simulink model "GasTurbine_Dyn_Template_GPT_RLS_Blocks"  (Simulink 9.2)
settings: Solver=ode4  StartTime=0.0  StopTime=MWS.in.SimTime  FixedStep=MWS.Solve.T  RelTol=1e-3  EnableMultiTasking=on
PreLoadFcn:
  | tmats_rls_setup;
values from neighbouring files (symbols this model uses):
  MWS = tmats_gpt_setup()    [run_tmats_gpt.m]
undefined symbols (not defined in the file or in its folder): RLS, stripchar_TMATS
libraries: simulink x7, Lib_Solve_ModelSource_TMATS x2, Lib_Cntrl_FirstOrderSensor_TMATS x1, Lib_Turbo_Ambient_TMATS x1, Lib_Turbo_Burner_TMATS x1, Lib_Turbo_Compressor_TMATS x1, Lib_Turbo_Duct_TMATS x1, Lib_Turbo_Inlet_TMATS x1, Lib_Turbo_Nozzle_TMATS x1, Lib_Turbo_Shaft_TMATS x1, Lib_Turbo_Turbine_TMATS x1, Lib_Solve_IterNRSolverJC_TMATS x1
Description:
  | Basic-block RLS ARX(5,5,1) fuel-to-acceleration observer. No estimator S-function or MATLAB Function.
settings Model: Creator=jwchapm2  LastModifiedBy=volka
settings DataIOCC: SignalLoggingSaveFormat=Dataset  SignalLoggingName=SimulationOutput
settings OptimizationCC: BlockReduction=off  DefaultParameterBehavior=Inlined  BufferReuse=off  ExpressionDepthLimit=2147483647
settings DebuggingCC: SolverPrmCheckMsg=warning  FcnCallInpInsideContextMsg=error
settings GRTTargetCC: CombineOutputUpdateFcns=on  GRTInterface=off

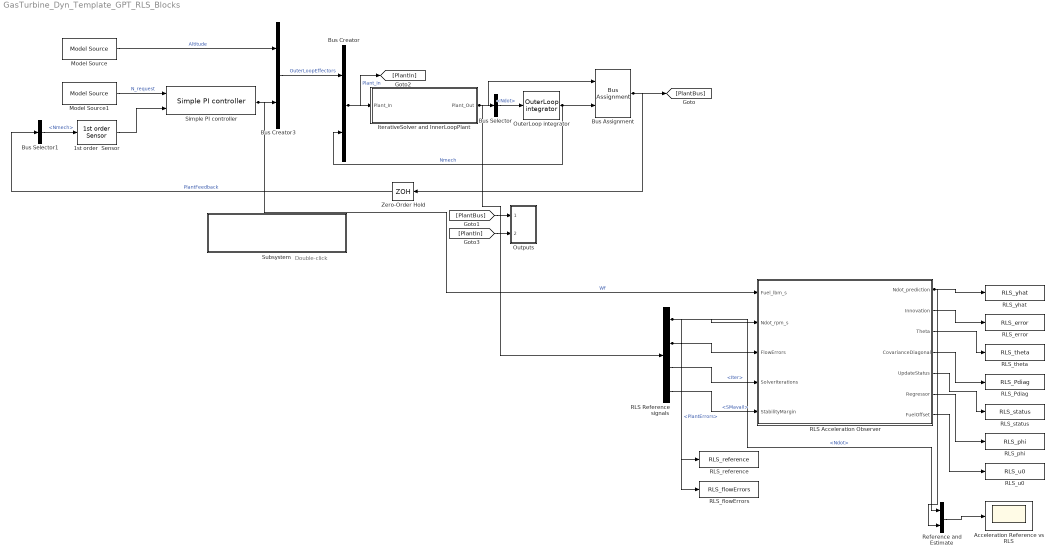
== system GasTurbine_Dyn_Template_GPT_RLS_Blocks ==
  note: Double-click
  1st order  Sensor : Lib_Cntrl_FirstOrderSensor_TMATS/1st order  Sensor  IC_M=MWS.Solve.N_IC  Sen_Max_M=20000  Sen_Min_M=0  Gain_M=1  Tau_M=0.05  GN_EN_M=off  GN_NST_M=MWS.Solve.T  GN_C_M=1  GN_MinNoise_M=0.3  F_Gain_M=1  F_Drift_M=0
  Acceleration Reference vs RLS : Scope
  Bus Assignment : BusAssignment  AssignedSignals=PlantBus.Nmech
  Bus Creator : BusCreator  Inputs=2
  Bus Creator3 : BusCreator  Inputs=2
  Bus Selector : BusSelector  OutputSignals=PlantBus.Ndot
  Bus Selector1 : BusSelector  OutputSignals=PlantBus.Nmech
  IterativeSolver and InnerLoopPlant : Subsystem
  Model Source : Lib_Solve_ModelSource_TMATS/Model Source  T_vec_M=MWS.in.t_vec  input_array_M=MWS.in.Alt
  Model Source1 : Lib_Solve_ModelSource_TMATS/Model Source  T_vec_M=MWS.in.t_vec  input_array_M=MWS.in.Ndmd
  OuterLoop integrator : Lib_Solve_OuterLoopIntegrator_TMATS/OuterLoop integrator  OL_IC_M=MWS.Solve.N_IC
  Outputs : Subsystem
  RLS Acceleration Observer : Subsystem
  RLS Reference signals : BusSelector  OutputSignals=PlantBus.Ndot,PlantErrors,PlantBus.Iter,PlantBus.C_Data.SMavail
  RLS_Pdiag : ToWorkspace  VariableName=RLS_Pdiag  SaveFormat=Timeseries  SampleTime=-1
  RLS_error : ToWorkspace  VariableName=RLS_error  SaveFormat=Timeseries  SampleTime=-1
  RLS_flowErrors : ToWorkspace  VariableName=RLS_flowErrors  SaveFormat=Timeseries  SampleTime=-1
  RLS_phi : ToWorkspace  VariableName=RLS_phi  SaveFormat=Timeseries  SampleTime=-1
  RLS_reference : ToWorkspace  VariableName=RLS_reference  SaveFormat=Timeseries  SampleTime=-1
  RLS_status : ToWorkspace  VariableName=RLS_status  SaveFormat=Timeseries  SampleTime=-1
  RLS_theta : ToWorkspace  VariableName=RLS_theta  SaveFormat=Timeseries  SampleTime=-1
  RLS_u0 : ToWorkspace  VariableName=RLS_u0  SaveFormat=Timeseries  SampleTime=-1
  RLS_yhat : ToWorkspace  VariableName=RLS_yhat  SaveFormat=Timeseries  SampleTime=-1
  Reference and Estimate : Mux  Inputs=2
  Simple PI controller : Lib_Cntrl_SimplePIcontroller_TMATS/Simple PI controller  Kp_M=0.05/2  Ki_M=0.1/2  PI_IC_M=3
  Subsystem : Subsystem
      settings: OpenFcn=run('PlotDynData.m')
      mask Display: fprintf('Plot Outputs')
  Zero-Order Hold : ZeroOrderHold  SampleTime=MWS.Solve.T
  wires:
  Bus Selector1/1 -> 1st order  Sensor/1  "<Nmech>"
  Reference and Estimate/1 -> Acceleration Reference vs RLS/1
  IterativeSolver and InnerLoopPlant/1(Plant_Out) -> Bus Assignment/1, Bus Selector/1, RLS Reference signals/1
  OuterLoop integrator/1 -> Bus Assignment/2, Bus Creator/2  "Nmech"
  Bus Creator3/1 -> Bus Creator/1  "OuterLoopEffectors"
  Model Source/1 -> Bus Creator3/1  "Altitude"
  Simple PI controller/1 -> Bus Creator3/2, RLS Acceleration Observer/1(Fuel_lbm_s)  "Wf"
  Zero-Order Hold/1 -> Bus Selector1/1  "PlantFeedback"
  Bus Assignment/1 -> [PlantBus], Zero-Order Hold/1
  Bus Creator/1 -> [PlantIn], IterativeSolver and InnerLoopPlant/1(Plant_In)  "Plant_In"
  Bus Selector/1 -> OuterLoop integrator/1  "<Ndot>"
  [PlantBus] -> Outputs/1(PlantOut)
  [PlantIn] -> Outputs/2(PlantIn)
  RLS Reference signals/1 -> RLS Acceleration Observer/2(Ndot_rpm_s), RLS_reference/1, Reference and Estimate/1  "<Ndot>"
  RLS Reference signals/2 -> RLS Acceleration Observer/3(FlowErrors), RLS_flowErrors/1  "<PlantErrors>"
  RLS Reference signals/3 -> RLS Acceleration Observer/4(SolverIterations)  "<Iter>"
  RLS Reference signals/4 -> RLS Acceleration Observer/5(StabilityMargin)  "<SMavail>"
  RLS Acceleration Observer/4(CovarianceDiagonal) -> RLS_Pdiag/1
  RLS Acceleration Observer/2(Innovation) -> RLS_error/1
  RLS Acceleration Observer/6(Regressor) -> RLS_phi/1
  RLS Acceleration Observer/5(UpdateStatus) -> RLS_status/1
  RLS Acceleration Observer/3(Theta) -> RLS_theta/1
  RLS Acceleration Observer/7(FuelOffset) -> RLS_u0/1
  RLS Acceleration Observer/1(Ndot_prediction) -> RLS_yhat/1, Reference and Estimate/2
  Model Source1/1 -> Simple PI controller/1  "N_request"
  1st order  Sensor/1 -> Simple PI controller/2

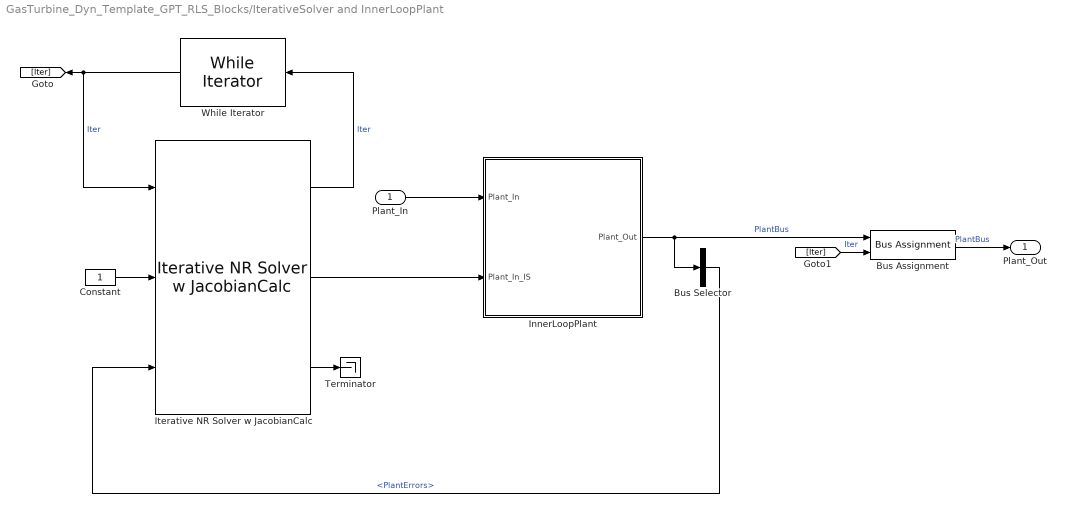
== system GasTurbine_Dyn_Template_GPT_RLS_Blocks/IterativeSolver and InnerLoopPlant ==
  Plant_In : Inport
  Bus Assignment : BusAssignment  AssignedSignals=PlantBus.Iter
  Bus Selector : BusSelector  OutputSignals=PlantErrors
  Constant : Constant
  InnerLoopPlant : Subsystem
  Iterative NR Solver w JacobianCalc : Lib_Solve_IterNRSolverJC_TMATS/Iterative NR Solver w JacobianCalc  SJac_Per_M=MWS.Solve.J_Calc_Per  SNR_IC_M=MWS.Solve.NR_IC  SNR_DX_M=MWS.Solve.NR_dx  SNR_Mx_M=100000  SNR_Mn_M=0.0001  SJacobianAttempts_M=MWS.Solve.NR_Jac_Re  Cond_Limits_M=MWS.Solve.C_Lim
  Terminator : Terminator
  While Iterator : WhileIterator  MaxIters=MWS.Solve.Max_Iter  WhileBlockType=do-while  ShowIterationPort=on
  Plant_Out : Outport
  wires:
  Plant_In/1 -> InnerLoopPlant/1(Plant_In)
  Bus Selector/1 -> Iterative NR Solver w JacobianCalc/3  "<PlantErrors>"
  While Iterator/1 -> [Iter], Iterative NR Solver w JacobianCalc/1  "Iter"
  InnerLoopPlant/1(Plant_Out) -> Bus Assignment/1, Bus Selector/1  "PlantBus"
  Iterative NR Solver w JacobianCalc/2 -> InnerLoopPlant/2(Plant_In_IS)
  Iterative NR Solver w JacobianCalc/1 -> While Iterator/1  "Iter"
  Iterative NR Solver w JacobianCalc/3 -> Terminator/1
  Constant/1 -> Iterative NR Solver w JacobianCalc/2
  [Iter] -> Bus Assignment/2  "Iter"
  Bus Assignment/1 -> Plant_Out/1  "PlantBus"

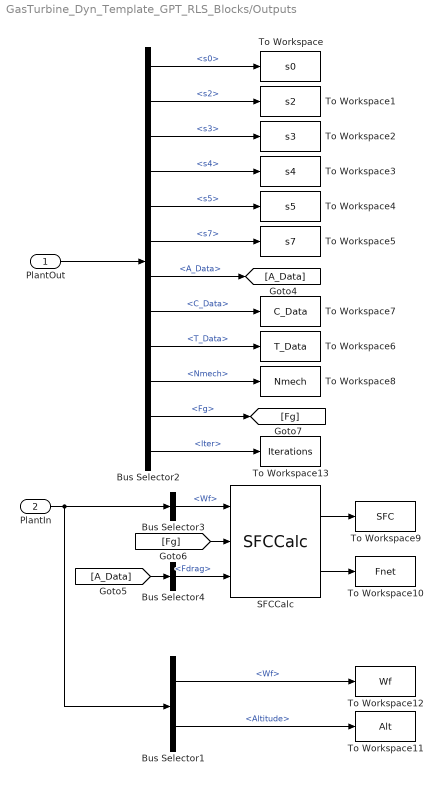
== system GasTurbine_Dyn_Template_GPT_RLS_Blocks/Outputs ==
  PlantOut : Inport
  PlantIn : Inport  Port=2
  Bus Selector1 : BusSelector  OutputSignals=OuterLoopEffectors.Wf,OuterLoopEffectors.Altitude
  Bus Selector2 : BusSelector  OutputSignals=PlantBus.s0,PlantBus.s2,PlantBus.s3,PlantBus.s4,PlantBus.s5,PlantBus.s7,PlantBus.A_Data,PlantBus.C_Data,PlantBus.T_Data,PlantBus.Nmech,PlantBus.Fg,PlantBus.Iter
  Bus Selector3 : BusSelector  OutputSignals=OuterLoopEffectors.Wf
  Bus Selector4 : BusSelector  OutputSignals=Fdrag
  SFCCalc : Lib_Turbo_SFCCalc_TMATS/SFCCalc
  To Workspace : ToWorkspace  VariableName=s0  SaveFormat=Timeseries  SampleTime=-1
  To Workspace1 : ToWorkspace  VariableName=s2  SaveFormat=Timeseries  SampleTime=-1
  To Workspace10 : ToWorkspace  VariableName=Fnet  SaveFormat=Timeseries  SampleTime=-1
  To Workspace11 : ToWorkspace  VariableName=Alt  SaveFormat=Timeseries  SampleTime=-1
  To Workspace12 : ToWorkspace  VariableName=Wf  SaveFormat=Timeseries  SampleTime=-1
  To Workspace13 : ToWorkspace  VariableName=Iterations  SaveFormat=Timeseries  SampleTime=-1
  To Workspace2 : ToWorkspace  VariableName=s3  SaveFormat=Timeseries  SampleTime=-1
  To Workspace3 : ToWorkspace  VariableName=s4  SaveFormat=Timeseries  SampleTime=-1
  To Workspace4 : ToWorkspace  VariableName=s5  SaveFormat=Timeseries  SampleTime=-1
  To Workspace5 : ToWorkspace  VariableName=s7  SaveFormat=Timeseries  SampleTime=-1
  To Workspace6 : ToWorkspace  VariableName=T_Data  SaveFormat=Timeseries  SampleTime=-1
  To Workspace7 : ToWorkspace  VariableName=C_Data  SaveFormat=Timeseries  SampleTime=-1
  To Workspace8 : ToWorkspace  VariableName=Nmech  SaveFormat=Timeseries  SampleTime=-1
  To Workspace9 : ToWorkspace  VariableName=SFC  SaveFormat=Timeseries  SampleTime=-1
  wires:
  SFCCalc/2 -> To Workspace10/1
  Bus Selector2/5 -> To Workspace4/1  "<s5>"
  SFCCalc/1 -> To Workspace9/1
  Bus Selector3/1 -> SFCCalc/1  "<Wf>"
  Bus Selector2/6 -> To Workspace5/1  "<s7>"
  Bus Selector2/11 -> [Fg]  "<Fg>"
  Bus Selector4/1 -> SFCCalc/3  "<Fdrag>"
  Bus Selector2/10 -> To Workspace8/1  "<Nmech>"
  Bus Selector2/1 -> To Workspace/1  "<s0>"
  Bus Selector2/3 -> To Workspace2/1  "<s3>"
  Bus Selector2/8 -> To Workspace7/1  "<C_Data>"
  Bus Selector2/9 -> To Workspace6/1  "<T_Data>"
  Bus Selector2/7 -> [A_Data]  "<A_Data>"
  PlantOut/1 -> Bus Selector2/1
  [Fg] -> SFCCalc/2
  Bus Selector2/2 -> To Workspace1/1  "<s2>"
  Bus Selector2/4 -> To Workspace3/1  "<s4>"
  PlantIn/1 -> Bus Selector1/1, Bus Selector3/1
  [A_Data] -> Bus Selector4/1
  Bus Selector1/1 -> To Workspace12/1  "<Wf>"
  Bus Selector1/2 -> To Workspace11/1  "<Altitude>"
  Bus Selector2/12 -> To Workspace13/1  "<Iter>"

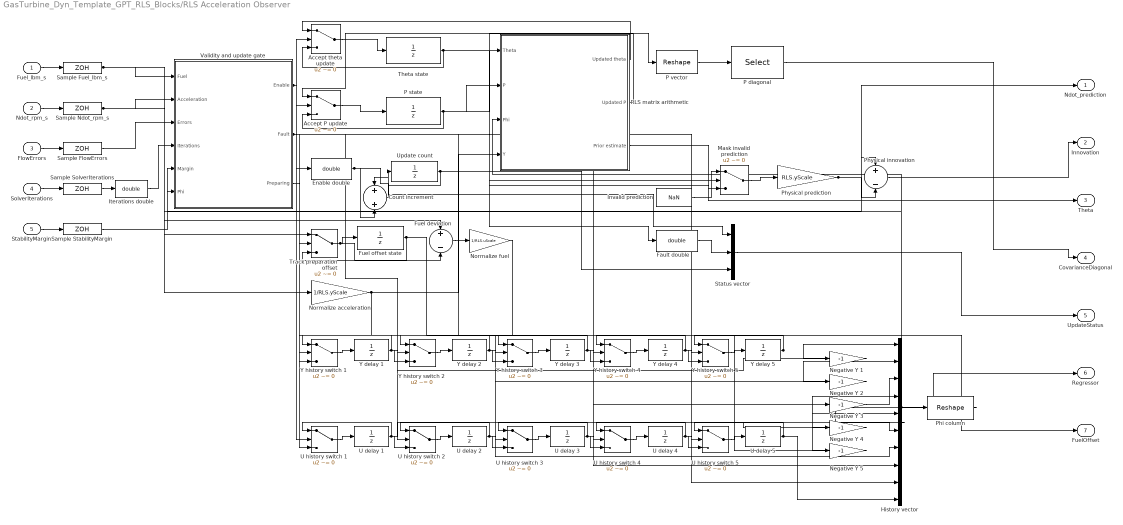
== system GasTurbine_Dyn_Template_GPT_RLS_Blocks/RLS Acceleration Observer ==
  Fuel_lbm_s : Inport
  Ndot_rpm_s : Inport  Port=2
  FlowErrors : Inport  Port=3
  SolverIterations : Inport  Port=4
  StabilityMargin : Inport  Port=5
  Accept P update : Switch  Criteria=u2 ~= 0
  Accept theta update : Switch  Criteria=u2 ~= 0
  Count increment : Sum
  Enable double : DataTypeConversion  OutDataTypeStr=double
  Fault double : DataTypeConversion  OutDataTypeStr=double
  Fuel deviation : Sum  Inputs=+-
  Fuel offset state : UnitDelay  InitialCondition=3  SampleTime=RLS.Ts
  History vector : Mux  Inputs=10
  Invalid prediction : Constant  Value=NaN
  Iterations double : DataTypeConversion  OutDataTypeStr=double
  Mask invalid prediction : Switch  Criteria=u2 ~= 0
  Negative Y {1..5} (5 alike) : Gain  Gain=-1
  Normalize acceleration : Gain  Gain=1/RLS.yScale
  Normalize fuel : Gain  Gain=1/RLS.uScale
  P diagonal : Selector  InputPortWidth=100  IndexOptions=Index vector (dialog)  Indices=1:11:100  OutputSizes=1
  P state : UnitDelay  InitialCondition=RLS.P0*eye(10)  SampleTime=RLS.Ts
  P vector : Reshape
  Phi column : Reshape  OutputDimensionality=Customize  OutputDimensions=[10 1]
  Physical innovation : Sum  Inputs=+-
  Physical prediction : Gain  Gain=RLS.yScale
  RLS matrix arithmetic : Subsystem
  Sample FlowErrors : ZeroOrderHold  SampleTime=RLS.Ts
  Sample Fuel_lbm_s : ZeroOrderHold  SampleTime=RLS.Ts
  Sample Ndot_rpm_s : ZeroOrderHold  SampleTime=RLS.Ts
  Sample SolverIterations : ZeroOrderHold  SampleTime=RLS.Ts
  Sample StabilityMargin : ZeroOrderHold  SampleTime=RLS.Ts
  Status vector : Mux  Inputs=3
  Theta state : UnitDelay  InitialCondition=zeros(10,1)  SampleTime=RLS.Ts
  Track preparation offset : Switch  Criteria=u2 ~= 0
  U delay {1..5} (5 alike) : UnitDelay  SampleTime=RLS.Ts
  U history switch {1..5} (5 alike) : Switch  Criteria=u2 ~= 0
  Update count : UnitDelay  SampleTime=RLS.Ts
  Validity and update gate : Subsystem
  Y delay {1..5} (5 alike) : UnitDelay  SampleTime=RLS.Ts
  Y history switch {1..5} (5 alike) : Switch  Criteria=u2 ~= 0
  Ndot_prediction : Outport
  Innovation : Outport  Port=2
  Theta : Outport  Port=3
  CovarianceDiagonal : Outport  Port=4
  UpdateStatus : Outport  Port=5
  Regressor : Outport  Port=6
  FuelOffset : Outport  Port=7
  wires:
  Fuel_lbm_s/1 -> Sample Fuel_lbm_s/1
  Ndot_rpm_s/1 -> Sample Ndot_rpm_s/1
  FlowErrors/1 -> Sample FlowErrors/1
  SolverIterations/1 -> Sample SolverIterations/1
  StabilityMargin/1 -> Sample StabilityMargin/1
  Sample SolverIterations/1 -> Iterations double/1
  Sample Fuel_lbm_s/1 -> Validity and update gate/1(Fuel), Track preparation offset/1, Fuel deviation/1
  Sample Ndot_rpm_s/1 -> Validity and update gate/2(Acceleration), Normalize acceleration/1, Physical innovation/1
  Sample FlowErrors/1 -> Validity and update gate/3(Errors)
  Iterations double/1 -> Validity and update gate/4(Iterations)
  Sample StabilityMargin/1 -> Validity and update gate/5(Margin)
  Validity and update gate/3(Preparing) -> Track preparation offset/2
  Fuel offset state/1 -> Track preparation offset/3, FuelOffset/1
  Track preparation offset/1 -> Fuel offset state/1, Fuel deviation/2
  Fuel deviation/1 -> Normalize fuel/1
  Y delay 1/1 -> Y history switch 1/1, Y history switch 2/3, Negative Y 1/1
  Validity and update gate/2(Fault) -> Y history switch 1/2, Y history switch 2/2, Y history switch 3/2, Y history switch 4/2, Y history switch 5/2, U history switch 1/2, U history switch 2/2, U history switch 3/2, U history switch 4/2, U history switch 5/2, Mask invalid prediction/2, Fault double/1
  Normalize acceleration/1 -> Y history switch 1/3, RLS matrix arithmetic/4(Y)
  Y history switch 1/1 -> Y delay 1/1
  Y delay 2/1 -> Y history switch 2/1, Y history switch 3/3, Negative Y 2/1
  Y history switch 2/1 -> Y delay 2/1
  Y delay 3/1 -> Y history switch 3/1, Y history switch 4/3, Negative Y 3/1
  Y history switch 3/1 -> Y delay 3/1
  Y delay 4/1 -> Y history switch 4/1, Y history switch 5/3, Negative Y 4/1
  Y history switch 4/1 -> Y delay 4/1
  Y delay 5/1 -> Y history switch 5/1, Negative Y 5/1
  Y history switch 5/1 -> Y delay 5/1
  U delay 1/1 -> U history switch 1/1, U history switch 2/3, History vector/6
  Normalize fuel/1 -> U history switch 1/3
  U history switch 1/1 -> U delay 1/1
  U delay 2/1 -> U history switch 2/1, U history switch 3/3, History vector/7
  U history switch 2/1 -> U delay 2/1
  U delay 3/1 -> U history switch 3/1, U history switch 4/3, History vector/8
  U history switch 3/1 -> U delay 3/1
  U delay 4/1 -> U history switch 4/1, U history switch 5/3, History vector/9
  U history switch 4/1 -> U delay 4/1
  U delay 5/1 -> U history switch 5/1, History vector/10
  U history switch 5/1 -> U delay 5/1
  Negative Y 1/1 -> History vector/1
  Negative Y 2/1 -> History vector/2
  Negative Y 3/1 -> History vector/3
  Negative Y 4/1 -> History vector/4
  Negative Y 5/1 -> History vector/5
  History vector/1 -> Phi column/1
  Phi column/1 -> Validity and update gate/6(Phi), RLS matrix arithmetic/3(Phi), Regressor/1
  Theta state/1 -> RLS matrix arithmetic/1(Theta), Accept theta update/3, Theta/1
  P state/1 -> RLS matrix arithmetic/2(P), Accept P update/3, P vector/1
  RLS matrix arithmetic/1(Updated theta) -> Accept theta update/1
  Validity and update gate/1(Enable) -> Accept theta update/2, Accept P update/2, Enable double/1
  RLS matrix arithmetic/2(Updated P) -> Accept P update/1
  Accept theta update/1 -> Theta state/1
  Accept P update/1 -> P state/1
  Invalid prediction/1 -> Mask invalid prediction/1
  RLS matrix arithmetic/3(Prior estimate) -> Mask invalid prediction/3
  Mask invalid prediction/1 -> Physical prediction/1
  Physical prediction/1 -> Physical innovation/2, Ndot_prediction/1
  P vector/1 -> P diagonal/1
  Update count/1 -> Count increment/1, Status vector/3
  Enable double/1 -> Count increment/2, Status vector/1
  Count increment/1 -> Update count/1
  Fault double/1 -> Status vector/2
  Physical innovation/1 -> Innovation/1
  P diagonal/1 -> CovarianceDiagonal/1
  Status vector/1 -> UpdateStatus/1

== system GasTurbine_Dyn_Template_GPT_RLS_Blocks/Subsystem ==

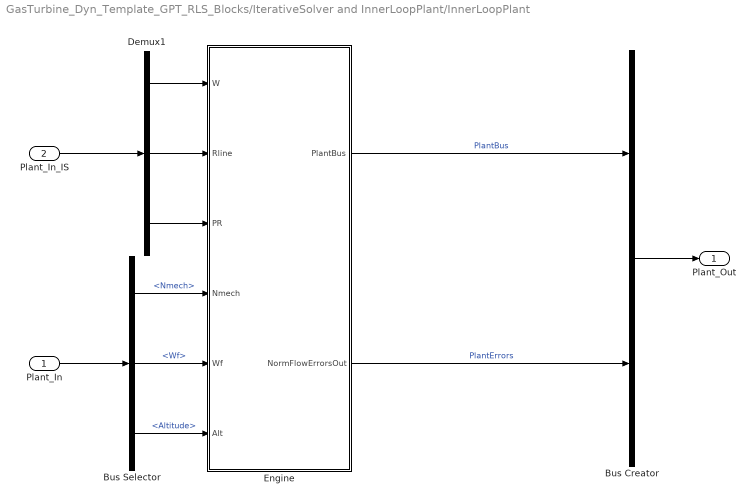
== system GasTurbine_Dyn_Template_GPT_RLS_Blocks/IterativeSolver and InnerLoopPlant/InnerLoopPlant ==
  Plant_In : Inport
  Plant_In_IS : Inport  Port=2
  Bus Selector : BusSelector  OutputSignals=Nmech,OuterLoopEffectors.Wf,OuterLoopEffectors.Altitude
  Bus Creator : BusCreator  Inputs=2
  Demux1 : Demux  Outputs=3
  Engine : Subsystem
  Plant_Out : Outport
  wires:
  Engine/1(PlantBus) -> Bus Creator/1  "PlantBus"
  Engine/2(NormFlowErrorsOut) -> Bus Creator/2  "PlantErrors"
  Bus Creator/1 -> Plant_Out/1
  Bus Selector/2 -> Engine/5(Wf)  "<Wf>"
  Bus Selector/1 -> Engine/4(Nmech)  "<Nmech>"
  Bus Selector/3 -> Engine/6(Alt)  "<Altitude>"
  Demux1/1 -> Engine/1(W)
  Demux1/2 -> Engine/2(Rline)
  Demux1/3 -> Engine/3(PR)
  Plant_In/1 -> Bus Selector/1
  Plant_In_IS/1 -> Demux1/1

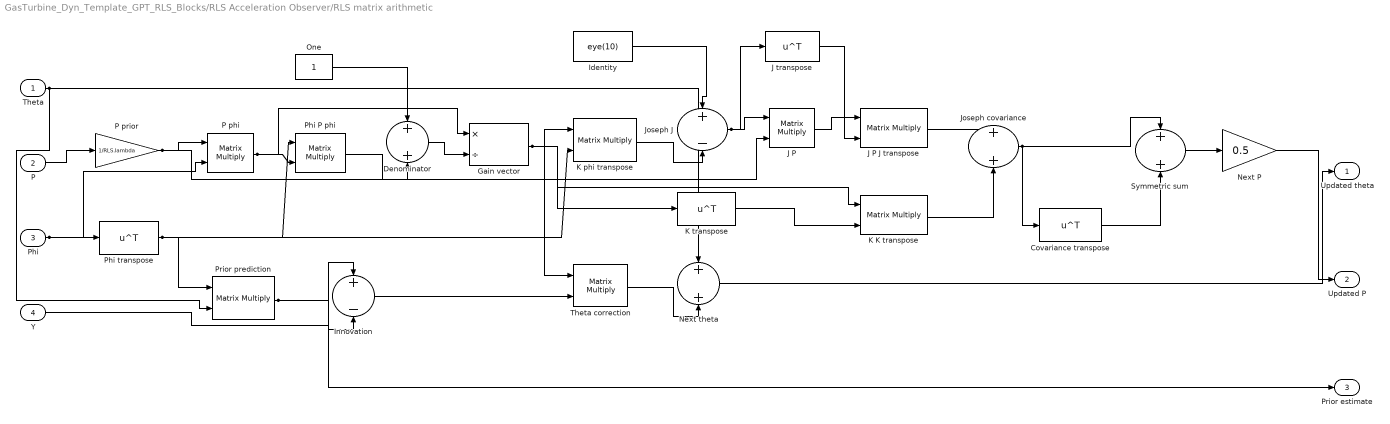
== system GasTurbine_Dyn_Template_GPT_RLS_Blocks/RLS Acceleration Observer/RLS matrix arithmetic ==
  Theta : Inport
  P : Inport  Port=2
  Phi : Inport  Port=3
  Y : Inport  Port=4
  Covariance transpose : Math  Operator=transpose  SaturateOnIntegerOverflow=on
  Denominator : Sum
  Gain vector : Product  Inputs=*/
  Identity : Constant  Value=eye(10)
  Innovation : Sum  Inputs=+-
  J P : Product  Inputs=**  Multiplication=Matrix(*)
  J P J transpose : Product  Inputs=**  Multiplication=Matrix(*)
  J transpose : Math  Operator=transpose  SaturateOnIntegerOverflow=on
  Joseph J : Sum  Inputs=+-
  Joseph covariance : Sum
  K K transpose : Product  Inputs=**  Multiplication=Matrix(*)
  K phi transpose : Product  Inputs=**  Multiplication=Matrix(*)
  K transpose : Math  Operator=transpose  SaturateOnIntegerOverflow=on
  Next P : Gain  Gain=0.5
  Next theta : Sum
  One : Constant
  P phi : Product  Inputs=**  Multiplication=Matrix(*)
  P prior : Gain  Gain=1/RLS.lambda
  Phi P phi : Product  Inputs=**  Multiplication=Matrix(*)
  Phi transpose : Math  Operator=transpose  SaturateOnIntegerOverflow=on
  Prior prediction : Product  Inputs=**  Multiplication=Matrix(*)
  Symmetric sum : Sum
  Theta correction : Product  Inputs=**  Multiplication=Matrix(*)
  Updated theta : Outport
  Updated P : Outport  Port=2
  Prior estimate : Outport  Port=3
  wires:
  P/1 -> P prior/1
  Phi/1 -> Phi transpose/1, P phi/2
  P prior/1 -> P phi/1, J P/2
  Phi transpose/1 -> Phi P phi/1, Prior prediction/1, K phi transpose/2
  P phi/1 -> Phi P phi/2, Gain vector/1
  One/1 -> Denominator/1
  Phi P phi/1 -> Denominator/2
  Denominator/1 -> Gain vector/2
  Theta/1 -> Prior prediction/2, Next theta/1
  Y/1 -> Innovation/1
  Prior prediction/1 -> Innovation/2, Prior estimate/1
  Gain vector/1 -> Theta correction/1, K phi transpose/1, K transpose/1, K K transpose/1
  Innovation/1 -> Theta correction/2
  Theta correction/1 -> Next theta/2
  Identity/1 -> Joseph J/1
  K phi transpose/1 -> Joseph J/2
  Joseph J/1 -> J P/1, J transpose/1
  J P/1 -> J P J transpose/1
  J transpose/1 -> J P J transpose/2
  K transpose/1 -> K K transpose/2
  J P J transpose/1 -> Joseph covariance/1
  K K transpose/1 -> Joseph covariance/2
  Joseph covariance/1 -> Covariance transpose/1, Symmetric sum/1
  Covariance transpose/1 -> Symmetric sum/2
  Symmetric sum/1 -> Next P/1
  Next theta/1 -> Updated theta/1
  Next P/1 -> Updated P/1

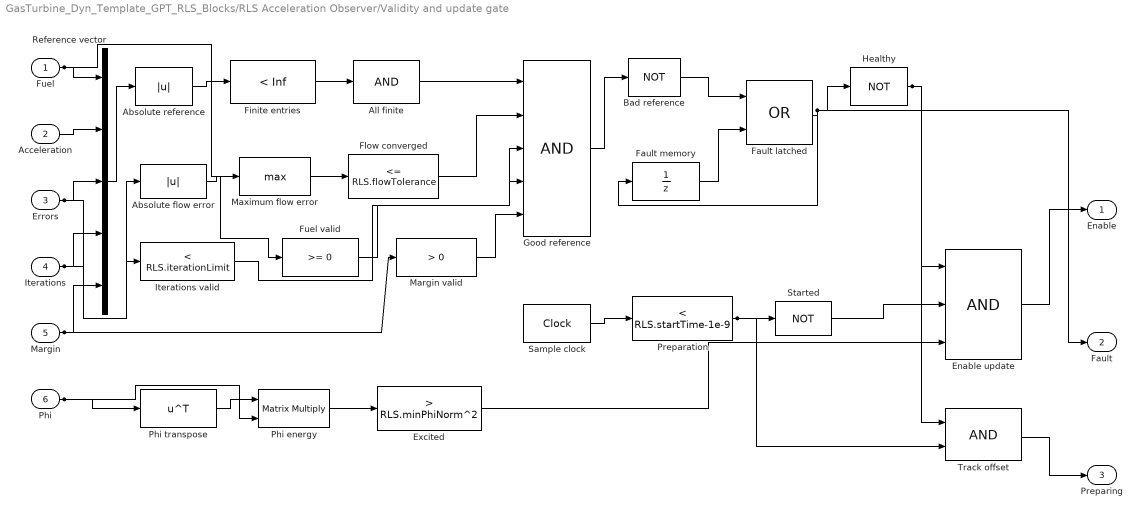
== system GasTurbine_Dyn_Template_GPT_RLS_Blocks/RLS Acceleration Observer/Validity and update gate ==
  Fuel : Inport
  Acceleration : Inport  Port=2
  Errors : Inport  Port=3
  Iterations : Inport  Port=4
  Margin : Inport  Port=5
  Phi : Inport  Port=6
  Absolute flow error : Abs
  Absolute reference : Abs
  All finite : Logic  Inputs=1  AllPortsSameDT=off  OutDataTypeStr=boolean
  Bad reference : Logic  Operator=NOT  AllPortsSameDT=off  OutDataTypeStr=boolean
  Enable update : Logic  Inputs=3  AllPortsSameDT=off  OutDataTypeStr=boolean
  Excited : simulink/Logic and Bit Operations/Compare To Constant  relop=>  const=RLS.minPhiNorm^2  OutDataTypeStr=boolean
  Fault latched : Logic  Operator=OR  AllPortsSameDT=off  OutDataTypeStr=boolean
  Fault memory : UnitDelay  InitialCondition=false  SampleTime=RLS.Ts
  Finite entries : simulink/Logic and Bit Operations/Compare To Constant  relop=<  const=Inf  OutDataTypeStr=boolean
  Flow converged : simulink/Logic and Bit Operations/Compare To Constant  relop=<=  const=RLS.flowTolerance  OutDataTypeStr=boolean
  Fuel valid : simulink/Logic and Bit Operations/Compare To Constant  relop=>=  const=0  OutDataTypeStr=boolean
  Good reference : Logic  Inputs=5  AllPortsSameDT=off  OutDataTypeStr=boolean
  Healthy : Logic  Operator=NOT  AllPortsSameDT=off  OutDataTypeStr=boolean
  Iterations valid : simulink/Logic and Bit Operations/Compare To Constant  relop=<  const=RLS.iterationLimit  OutDataTypeStr=boolean
  Margin valid : simulink/Logic and Bit Operations/Compare To Constant  relop=>  const=0  OutDataTypeStr=boolean
  Maximum flow error : MinMax  Function=max
  Phi energy : Product  Inputs=**  Multiplication=Matrix(*)
  Phi transpose : Math  Operator=transpose  SaturateOnIntegerOverflow=on
  Preparation : simulink/Logic and Bit Operations/Compare To Constant  relop=<  const=RLS.startTime-1e-9  OutDataTypeStr=boolean
  Reference vector : Mux  Inputs=5
  Sample clock : DigitalClock  SampleTime=RLS.Ts
  Started : Logic  Operator=NOT  AllPortsSameDT=off  OutDataTypeStr=boolean
  Track offset : Logic  AllPortsSameDT=off  OutDataTypeStr=boolean
  Enable : Outport
  Fault : Outport  Port=2
  Preparing : Outport  Port=3
  wires:
  Fuel/1 -> Reference vector/1, Fuel valid/1
  Acceleration/1 -> Reference vector/2
  Errors/1 -> Reference vector/3, Absolute flow error/1
  Iterations/1 -> Reference vector/4, Iterations valid/1
  Margin/1 -> Reference vector/5, Margin valid/1
  Reference vector/1 -> Absolute reference/1
  Absolute reference/1 -> Finite entries/1
  Finite entries/1 -> All finite/1
  Absolute flow error/1 -> Maximum flow error/1
  Maximum flow error/1 -> Flow converged/1
  All finite/1 -> Good reference/1
  Flow converged/1 -> Good reference/2
  Iterations valid/1 -> Good reference/3
  Fuel valid/1 -> Good reference/4
  Margin valid/1 -> Good reference/5
  Good reference/1 -> Bad reference/1
  Bad reference/1 -> Fault latched/1
  Fault memory/1 -> Fault latched/2
  Fault latched/1 -> Fault memory/1, Healthy/1, Fault/1
  Sample clock/1 -> Preparation/1
  Preparation/1 -> Started/1, Track offset/2
  Phi/1 -> Phi transpose/1, Phi energy/2
  Phi transpose/1 -> Phi energy/1
  Phi energy/1 -> Excited/1
  Healthy/1 -> Enable update/1, Track offset/1
  Started/1 -> Enable update/2
  Excited/1 -> Enable update/3
  Enable update/1 -> Enable/1
  Track offset/1 -> Preparing/1

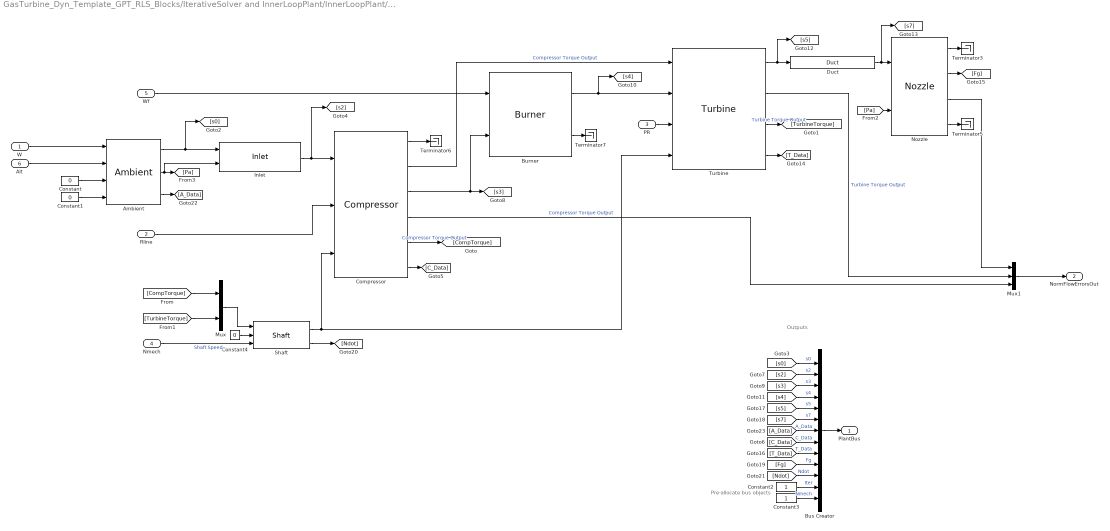
== system GasTurbine_Dyn_Template_GPT_RLS_Blocks/IterativeSolver and InnerLoopPlant/InnerLoopPlant/Engine ==
  note: Pre-allocate bus objects
  note: Outputs
  W : Inport
  Rline : Inport  Port=2
  PR : Inport  Port=3
  Nmech : Inport  Port=4
  Wf : Inport  Port=5
  Alt : Inport  Port=6
  Ambient : Lib_Turbo_Ambient_TMATS/Ambient  X_A_AltVec_M=5000*[-1 0 1 2 3 4 5 6 7 8 9 10 12 14 16]  T_A_TsVec_M=[536.51 518.67 500.84 483.03 465.22 447.41 429.62 411.84 394.06 389.97 389.97 389.97 389.97 392.25 397.69]  T_A_PsVec_M=[17.554 14.696 12.228 10.108 8.297 6.759 5.461 4.373 3.468 2.73 2.149 1.692 1.049 0.651 0.406]  AFARc_M=0  X_A_FARVec_M=[0; 0.0050; 0.0100; 0.0150; 0.0200; 0.0250; 0.0300]  T_A_RtArray_M="[0.0686;    0.0686;    0.0686;    0.0686;    0.0686;    0.0686;    0.0686]"  Y_A_TVec_M=[300 10000]  T_A_gammaArray_M=[ 1.4 1.4 1.4 1.4 1.4 1.4 1.4; 1.4 1.4 1.4 1.4 1.4 1.4 1.4]
  Burner : Lib_Turbo_Burner_TMATS/Burner  LHVEn_M=on  LHV_M=MWS.Burner.LHV  Eff_M=1  hFuel_M=-1200  dPnormBurner_M=MWS.Burner.dP
  Bus Creator : BusCreator  Inputs=13
  Compressor : Lib_Turbo_Compressor_TMATS/Compressor  X_C_RlineVec_M=MWS.HPC.RlineVec  Z_C_AlphaVec_M=1  Y_C_Map_NcVec_M=MWS.HPC.NcVec  T_C_Map_WcArray_M=MWS.HPC.WcArray  T_C_Map_PRArray_M=MWS.HPC.PRArray  T_C_Map_EffArray_M=MWS.HPC.EffArray  s_C_Nc_M=MWS.HPC.s_Nc  s_C_Wc_M=MWS.HPC.s_Wc  s_C_PR_M=MWS.HPC.s_PR  s_C_Eff_M=MWS.HPC.s_eff  SL_M=off  Scale_M=none  CBLDEN_M=off  C_CBD_M=0  C_CBFht_M=0.5  C_CBFPt_M=0.5  FBLDEN_M=off  C_FBD_M=0  C_BFht_M=0.5  C_BFPt_M=0.5  DefSMEn_M=off  SMNEn_M=off  SRline_M=1  X_C_Map_WcSurgeVec_M=MWS.HPC.WcMapSurge  T_C_Map_PRSurgeVec_M=MWS.HPC.PRMapSurge  iDesign_M=2  NcDes_M=10000  EffDes_M=0.85  PRDes_M=20  RlineDes_M=2  FVar_M=strcat('iDes_',stripchar_TMATS(gcb),'.bin')  BlkNm_M=double(gcb)  HP_M=off
  Constant : Constant  Value=0
  Constant1 : Constant  Value=0
  Constant2 : Constant  OutDataTypeStr=int32
  Constant3 : Constant
  Constant4 : Constant  Value=0
  Duct : Lib_Turbo_Duct_TMATS/Duct  dP_M=MWS.Duct.dP
  Inlet : Lib_Turbo_Inlet_TMATS/Inlet  eRambase_M=MWS.Inlet.eRambase  X_eRamVec_M=[0 3]  T_eRamtbl_M=[1 1]
  Mux : Mux  Inputs=2
  Mux1 : Mux  Inputs=3
  Nozzle : Lib_Turbo_Nozzle_TMATS/Nozzle  SWType_M=Convergent  N_TArea_M=MWS.Noz.ATh  N_EArea_M=110.7  N_FL_M=MWS.Noz.LossPerc  X_N_TtVec2_M=MWS.Noz.TtVec  T_N_TGArray_M=MWS.Noz.TGArray  X_N_PEQPaVec_M=MWS.Noz.PeQPaVec  T_N_CdThArray_M=MWS.Noz.CdThArray  T_N_CvArray_M=MWS.Noz.CvArray  CfgEn_M=off  T_N_CfgArray_M=[1 1]  X_N_FARVec_M=MWS.Noz.FARVec  T_N_RtArray_M=MWS.Noz.RArray  Y_N_TtVec_M=MWS.Noz.TtVec  T_N_MAP_gammaArray_M=MWS.Noz.GArray  iDesign_M=2  WDes_M=100  FVar_M=strcat('iDes_',stripchar_TMATS(gcb),'.bin')
  Shaft : Lib_Turbo_Shaft_TMATS/Shaft  Shaft_Inertia_M=MWS.Shaft.N_I
  Terminator{3,5..7} (4 alike) : Terminator
  Turbine : Lib_Turbo_Turbine_TMATS/Turbine  X_T_Map_PRVec_M=MWS.HPT.PRVec  Y_T_Map_NcVec_M=MWS.HPT.NcVec  T_T_Map_WcArray_M=MWS.HPT.WcArray  T_T_Map_EffArray_M=MWS.HPT.EffArray  s_T_Nc_M=MWS.HPT.s_Nc  s_T_Wc_M=MWS.HPT.s_Wc  s_T_PR_M=MWS.HPT.s_PR  s_T_Eff_M=MWS.HPT.s_eff  ConfigNPSS_M=0  Scale_M=none  CFlwEn_M=off  T_CoolFlwPos_M=0  iDesign_M=2  NcDes_M=100  EffDes_M=0.9200  PRDes_M=5  NDes_M=10000  FVar_M=strcat('iDes_',stripchar_TMATS(gcb),'.bin')  BlkNm_M=double(gcb)  HP_M=off
  PlantBus : Outport
  NormFlowErrorsOut : Outport  Port=2
  wires:
  Compressor/6 -> [C_Data]
  Ambient/1 -> [s0], Inlet/1
  Duct/1 -> [s7], Nozzle/1
  Ambient/3 -> [A_Data]
  Ambient/2 -> [Pa], Inlet/2
  Constant1/1 -> Ambient/4
  Constant/1 -> Ambient/3
  W/1 -> Ambient/1
  Nozzle/2 -> [Fg]
  Compressor/2 -> Turbine/1  "Compressor Torque Output"
  Compressor/1 -> Terminator6/1
  Shaft/1 -> Compressor/3, Turbine/4
  [TurbineTorque] -> Mux/2
  [CompTorque] -> Mux/1
  Turbine/3 -> [TurbineTorque]  "Turbine Torque Output"
  Compressor/5 -> [CompTorque]  "Compressor Torque Output"
  Mux/1 -> Shaft/1
  Shaft/2 -> [Ndot]
  Nmech/1 -> Shaft/3  "Shaft Speed"
  Inlet/1 -> [s2], Compressor/1
  Alt/1 -> Ambient/2
  Compressor/4 -> Mux1/3  "Compressor Torque Output"
  Turbine/2 -> Mux1/2  "Turbine Torque Output"
  Nozzle/4 -> Terminator5/1
  Nozzle/3 -> Mux1/1
  Nozzle/1 -> Terminator3/1
  Turbine/4 -> [T_Data]
  Mux1/1 -> NormFlowErrorsOut/1
  Rline/1 -> Compressor/2
  PR/1 -> Turbine/3
  Turbine/1 -> [s5], Duct/1
  Burner/1 -> [s4], Turbine/2
  [Pa] -> Nozzle/2
  Burner/2 -> Terminator7/1
  Wf/1 -> Burner/1
  Compressor/3 -> [s3], Burner/2
  [s0] -> Bus Creator/1  "s0"
  [s2] -> Bus Creator/2  "s2"
  [s3] -> Bus Creator/3  "s3"
  [s4] -> Bus Creator/4  "s4"
  [s5] -> Bus Creator/5  "s5"
  [s7] -> Bus Creator/6  "s7"
  [C_Data] -> Bus Creator/8  "C_Data"
  [T_Data] -> Bus Creator/9  "T_Data"
  [Fg] -> Bus Creator/10  "Fg"
  [Ndot] -> Bus Creator/11  "Ndot"
  Bus Creator/1 -> PlantBus/1
  [A_Data] -> Bus Creator/7  "A_Data"
  Constant2/1 -> Bus Creator/12  "Iter"
  Constant3/1 -> Bus Creator/13  "Nmech"
  Constant4/1 -> Shaft/2
